simulink model "Md61Md62CalibSet"  (R2018b)
settings: Solver=FixedStepDiscrete  StartTime=0.0  StopTime=10.0  FixedStep=0.01  RelTol=1e-3
undefined symbols (not defined in the file or in its folder): KeSMSuFirstRwStBackPosDelta_Val, KeSMSuFirstRwStCushFoldPosDelta_Val, KeSMSuFirstRwStFwdBkwdPosDelta_Val, KeSMSuThrdRwCushFoldPosDelta_Val, KeSMSwAcsMd30PassStBkReclnUpwdDnwdPos1_Val, KeSMSwAcsMd30PassStBkReclnUpwdDnwdPos1Max_Val, KeSMSwAcsMd30PassStBkReclnUpwdDnwdPos1Min_Val, KeSMSwAcsMd30PassStFldUpwdDnwdPos1_Val, KeSMSwAcsMd30PassStFrwdBkwdPos1_Val, KeSMSwAcsMd30PassStFrwdBkwdPos1Max_Val, KeSMSwAcsMd30PassStFrwdBkwdPos1Min_Val, KeSMSwSeatBkLimitPos_Val, KeSMSwSeatBkLimitPosDelt_Val
libraries: StIsPosChkLib x2
(part 1 of 5)
settings Model: Creator=sn2xws  LastModifiedBy=sn55gm
settings Model: ModifiedHistory=|
  | 25.7.2 V3.13.0 新增Md61 Md62
  | 25.7.28 V3.13.1 BUG 1097903
  | 25.11.04 V3.13.2 副驾发送目标位置删除关于目标位置和limit的判断
settings DataIOCC: SaveFormat=StructureWithTime
settings OptimizationCC: DefaultParameterBehavior=Inlined  EnhancedBackFolding=on  PassReuseOutputArgsAs=Individual arguments  ZeroExternalMemoryAtStartup=off  ZeroInternalMemoryAtStartup=off  OptimizeBlockOrder=speed  DifferentSizesBufferReuse=on  OptimizationCustomize=off
settings DebuggingCC: ParameterTunabilityLossMsg=error
settings SFSimCC: MATLABDynamicMemAlloc=off
settings RTWCC: SystemTargetFile=autosar.tlc  GenCodeOnly=on  TemplateMakefile=ert_default_tmf  Description=AUTOSAR  GenerateReport=on  IncludeHyperlinkInReport=on  LaunchReport=on  GenerateTraceInfo=on  GenerateTraceReport=on  GenerateTraceReportSl=on  GenerateTraceReportSf=on  GenerateTraceReportEml=on
settings CodeAppCC: ForceParamTrailComments=on  IgnoreCustomStorageClasses=off  OperatorAnnotations=on  SimulinkDataObjDesc=on  SFDataObjDesc=on  InsertBlockDesc=on
settings STFCustomTargetCC: TargetLangStandard=C99 (ISO)  MultiwordLength=256  ParMdlRefBuildCompliant=on  CompOptLevelCompliant=on  IncludeMdlTerminateFcn=off  CombineOutputUpdateFcns=on  SuppressErrorStatus=on  ERTCustomFileBanners=on  SupportNonFinite=off  SupportComplex=off  SupportContinuousTime=off  SupportNonInlinedSFcns=off  RemoveResetFunc=on  MATLABClassNameForMDSCustomization=Simulink.SoftwareTarget.ERTCustomization  AutosarCompliant=on  UseToolchainInfoCompliant=on  LookupTableObjectStructAxisOrder=2,1,3,4,...  LUTObjectStructOrderEvenSpacing=Size,Table,Breakpoints  SystemTargetFile=autosar.tlc
settings ERTTargetCC: TargetLangStandard=C99 (ISO)  ConcurrentExecutionCompliant=off  IncludeMdlTerminateFcn=off  SuppressErrorStatus=on  SupportNonFinite=off  SupportComplex=off  ModelStepFunctionPrototypeControlCompliant=off  CPPClassGenCompliant=off  AutosarCompliant=on  LookupTableObjectStructAxisOrder=2,1,3,4,...  LUTObjectStructOrderEvenSpacing=Size,Table,Breakpoints  InlinedParameterPlacement=NonHierarchical  ERTCustomFileTemplate=example_file_process.tlc  ERTFilePackagingFormat=Compact

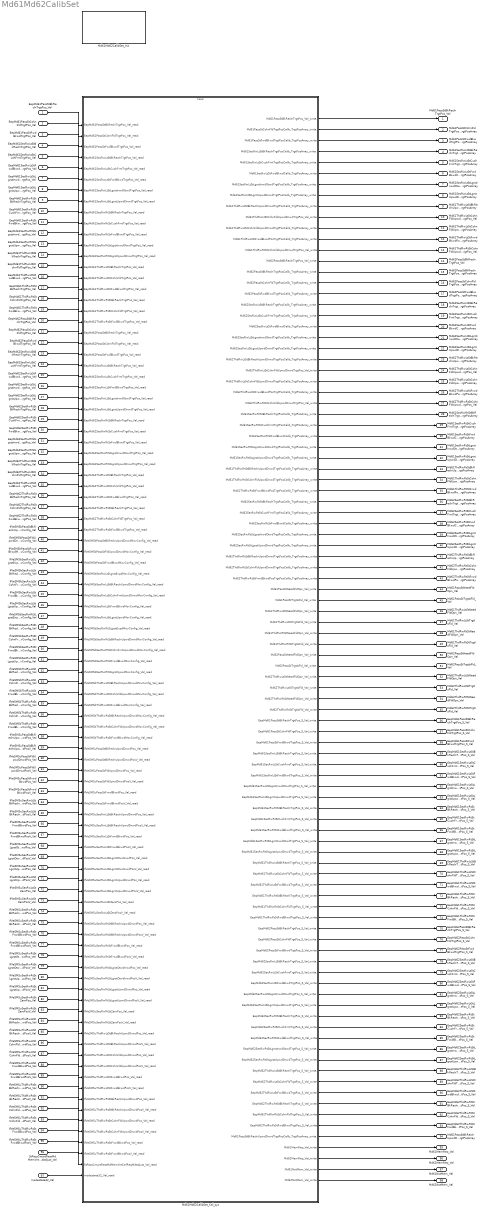
== system Md61Md62CalibSet ==
  EepMd61PassStBkReclnTrgtPos_Val : Inport  OutDataTypeStr=uint16  PortDimensions=1
  EepMd61PassStCshnFldTrgtPos_Val : Inport  Port=2  OutDataTypeStr=uint16  PortDimensions=1
  EepMd61PassStFwdBkwdTrgtPos_Val : Inport  Port=3  OutDataTypeStr=uint16  PortDimensions=1
  EepMd61SecRwLtStBkReclnTrgtPos_Val : Inport  Port=4  OutDataTypeStr=uint16  PortDimensions=1
  EepMd61SecRwLtStCushFrntTrgtPos_Val : Inport  Port=5  OutDataTypeStr=uint16  PortDimensions=1
  EepMd61SecRwLtStFwdBkwdTrgtPos_Val : Inport  Port=6  OutDataTypeStr=uint16  PortDimensions=1
  EepMd61SecRwLtStLgrstInwdOtwdTrgtPos_Val : Inport  Port=7  OutDataTypeStr=uint16  PortDimensions=1
  EepMd61SecRwLtStLgrstUpwdDnwdTrgtPos_Val : Inport  Port=8  OutDataTypeStr=uint16  PortDimensions=1
  EepMd61SecRwRtStBkReclnTrgtPos_Val : Inport  Port=9  OutDataTypeStr=uint16  PortDimensions=1
  EepMd61SecRwRtStCushFrntTrgtPos_Val : Inport  Port=10  OutDataTypeStr=uint16  PortDimensions=1
  EepMd61SecRwRtStFwdBkwdTrgtPos_Val : Inport  Port=11  OutDataTypeStr=uint16  PortDimensions=1
  EepMd61SecRwRtStLgrstInwdOtwdTrgtPos_Val : Inport  Port=12  OutDataTypeStr=uint16  PortDimensions=1
  EepMd61SecRwRtStLgrstUpwdDnwdTrgtPos_Val : Inport  Port=13  OutDataTypeStr=uint16  PortDimensions=1
  EepMd61ThdRwLtStBkReclnTrgtPos_Val : Inport  Port=14  OutDataTypeStr=uint16  PortDimensions=1
  EepMd61ThdRwLtStCshnFldTrgtPos_Val : Inport  Port=15  OutDataTypeStr=uint16  PortDimensions=1
  EepMd61ThdRwLtStFwdBkwdTrgtPos_Val : Inport  Port=16  OutDataTypeStr=uint16  PortDimensions=1
  EepMd61ThdRwRtStBkReclnTrgtPos_Val : Inport  Port=17  OutDataTypeStr=uint16  PortDimensions=1
  EepMd61ThdRwRtStCshnFldTrgtPos_Val : Inport  Port=18  OutDataTypeStr=uint16  PortDimensions=1
  EepMd61ThdRwRtStFwdBkwdTrgtPos_Val : Inport  Port=19  OutDataTypeStr=uint16  PortDimensions=1
  EepMd62PassStBkReclnTrgtPos_Val : Inport  Port=20  OutDataTypeStr=uint16  PortDimensions=1
  EepMd62PassStCshnFldTrgtPos_Val : Inport  Port=21  OutDataTypeStr=uint16  PortDimensions=1
  EepMd62PassStFwdBkwdTrgtPos_Val : Inport  Port=22  OutDataTypeStr=uint16  PortDimensions=1
  EepMd62SecRwLtStBkReclnTrgtPos_Val : Inport  Port=23  OutDataTypeStr=uint16  PortDimensions=1
  EepMd62SecRwLtStCushFrntTrgtPos_Val : Inport  Port=24  OutDataTypeStr=uint16  PortDimensions=1
  EepMd62SecRwLtStFwdBkwdTrgtPos_Val : Inport  Port=25  OutDataTypeStr=uint16  PortDimensions=1
  EepMd62SecRwLtStLgrstInwdOtwdTrgtPos_Val : Inport  Port=26  OutDataTypeStr=uint16  PortDimensions=1
  EepMd62SecRwLtStLgrstUpwdDnwdTrgtPos_Val : Inport  Port=27  OutDataTypeStr=uint16  PortDimensions=1
  EepMd62SecRwRtStBkReclnTrgtPos_Val : Inport  Port=28  OutDataTypeStr=uint16  PortDimensions=1
  EepMd62SecRwRtStCushFrntTrgtPos_Val : Inport  Port=29  OutDataTypeStr=uint16  PortDimensions=1
  EepMd62SecRwRtStFwdBkwdTrgtPos_Val : Inport  Port=30  OutDataTypeStr=uint16  PortDimensions=1
  EepMd62SecRwRtStLgrstInwdOtwdTrgtPos_Val : Inport  Port=31  OutDataTypeStr=uint16  PortDimensions=1
  EepMd62SecRwRtStLgrstUpwdDnwdTrgtPos_Val : Inport  Port=32  OutDataTypeStr=uint16  PortDimensions=1
  EepMd62ThdRwLtStBkReclnTrgtPos_Val : Inport  Port=33  OutDataTypeStr=uint16  PortDimensions=1
  EepMd62ThdRwLtStCshnFldTrgtPos_Val : Inport  Port=34  OutDataTypeStr=uint16  PortDimensions=1
  EepMd62ThdRwLtStFwdBkwdTrgtPos_Val : Inport  Port=35  OutDataTypeStr=uint16  PortDimensions=1
  EepMd62ThdRwRtStBkReclnTrgtPos_Val : Inport  Port=36  OutDataTypeStr=uint16  PortDimensions=1
  EepMd62ThdRwRtStCshnFldTrgtPos_Val : Inport  Port=37  OutDataTypeStr=uint16  PortDimensions=1
  EepMd62ThdRwRtStFwdBkwdTrgtPos_Val : Inport  Port=38  OutDataTypeStr=uint16  PortDimensions=1
  IfVeSMSbPassStBkReclnUpwdDnwdMovConfig_Val : Inport  Port=39  OutDataTypeStr=boolean  PortDimensions=1
  IfVeSMSbPassStFldUpwdDnwdMovConfig_Val : Inport  Port=40  OutDataTypeStr=boolean  PortDimensions=1
  IfVeSMSbPassStFrwdBkwdMovConfig_Val : Inport  Port=41  OutDataTypeStr=boolean  PortDimensions=1
  IfVeSMSbSecRwLtSLgrstExpdMovConfig_Val : Inport  Port=42  OutDataTypeStr=boolean  PortDimensions=1
  IfVeSMSbSecRwLtStBkReclnUpwdDnwdMovConfig_Val : Inport  Port=43  OutDataTypeStr=boolean  PortDimensions=1
  IfVeSMSbSecRwLtStCshnFrntUpwdDnwdMovConfig_Val : Inport  Port=44  OutDataTypeStr=boolean  PortDimensions=1
  IfVeSMSbSecRwLtStFrwdBkwdMovConfig_Val : Inport  Port=45  OutDataTypeStr=boolean  PortDimensions=1
  IfVeSMSbSecRwLtStLgrstUpwdMovConfig_Val : Inport  Port=46  OutDataTypeStr=boolean  PortDimensions=1
  IfVeSMSbSecRwRtSLgrstExpdMovConfig_Val : Inport  Port=47  OutDataTypeStr=boolean  PortDimensions=1
  IfVeSMSbSecRwRtStBkReclnUpwdDnwdMovConfig_Val : Inport  Port=48  OutDataTypeStr=boolean  PortDimensions=1
  IfVeSMSbSecRwRtStCshnFrntUpwdDnwdMovConfig_Val : Inport  Port=49  OutDataTypeStr=boolean  PortDimensions=1
  IfVeSMSbSecRwRtStFrwdBkwdMovConfig_Val : Inport  Port=50  OutDataTypeStr=boolean  PortDimensions=1
  IfVeSMSbSecRwRtStLgrstUpwdMovConfig_Val : Inport  Port=51  OutDataTypeStr=boolean  PortDimensions=1
  IfVeSMSbThdRwLtStBkReclnUpwdDnwdMovConfig_Val : Inport  Port=52  OutDataTypeStr=boolean  PortDimensions=1
  IfVeSMSbThdRwLtStCshnFldUpwdDnwdMovConfig_Val : Inport  Port=53  OutDataTypeStr=boolean  PortDimensions=1
  IfVeSMSbThdRwLtStFrwdBkwdMovConfig_Val : Inport  Port=54  OutDataTypeStr=boolean  PortDimensions=1
  IfVeSMSbThdRwRtStBkReclnUpwdDnwdMovConfig_Val : Inport  Port=55  OutDataTypeStr=boolean  PortDimensions=1
  IfVeSMSbThdRwRtStCshnFldUpwdDnwdMovConfig_Val : Inport  Port=56  OutDataTypeStr=boolean  PortDimensions=1
  IfVeSMSbThdRwRtStFrwdBkwdMovConfig_Val : Inport  Port=57  OutDataTypeStr=boolean  PortDimensions=1
  IfVeSMSuPassStBkReclnUpwdDnwdPos_Val : Inport  Port=58  OutDataTypeStr=uint16  PortDimensions=1
  IfVeSMSuPassStBkReclnUpwdDnwdPosV_Val : Inport  Port=59  OutDataTypeStr=boolean  PortDimensions=1
  IfVeSMSuPassStFldUpwdDnwdPos_Val : Inport  Port=60  OutDataTypeStr=uint16  PortDimensions=1
  IfVeSMSuPassStFldUpwdDnwdPosV_Val : Inport  Port=61  OutDataTypeStr=boolean  PortDimensions=1
  IfVeSMSuPassStFrwdBkwdPos_Val : Inport  Port=62  OutDataTypeStr=uint16  PortDimensions=1
  IfVeSMSuPassStFrwdBkwdPosV_Val : Inport  Port=63  OutDataTypeStr=boolean  PortDimensions=1
  IfVeSMSuSecRwLtStBkReclnUpwdDnwdPos_Val : Inport  Port=64  OutDataTypeStr=uint16  PortDimensions=1
  IfVeSMSuSecRwLtStBkReclnUpwdDnwdPosV_Val : Inport  Port=65  OutDataTypeStr=boolean  PortDimensions=1
  IfVeSMSuSecRwLtStFrwdBkwdPos_Val : Inport  Port=66  OutDataTypeStr=uint16  PortDimensions=1
  IfVeSMSuSecRwLtStFrwdBkwdPosV_Val : Inport  Port=67  OutDataTypeStr=boolean  PortDimensions=1
  IfVeSMSuSecRwLtStLgrstOtwdInwdPos_Val : Inport  Port=68  OutDataTypeStr=uint16  PortDimensions=1
  IfVeSMSuSecRwLtStLgrstOtwdInwdPosV_Val : Inport  Port=69  OutDataTypeStr=boolean  PortDimensions=1
  IfVeSMSuSecRwLtStLgrstUpwdDnwdPos_Val : Inport  Port=70  OutDataTypeStr=uint16  PortDimensions=1
  IfVeSMSuSecRwLtStLgrstUpwdDnwdPosV_Val : Inport  Port=71  OutDataTypeStr=boolean  PortDimensions=1
  IfVeSMSuSecRwLtStZeroPos_Val : Inport  Port=72  OutDataTypeStr=uint16  PortDimensions=1
  IfVeSMSuSecRwLtStZeroPosV_Val : Inport  Port=73  OutDataTypeStr=boolean  PortDimensions=1
  IfVeSMSuSecRwRtStBkReclnUpwdDnwdPos_Val : Inport  Port=74  OutDataTypeStr=uint16  PortDimensions=1
  IfVeSMSuSecRwRtStBkReclnUpwdDnwdPosV_Val : Inport  Port=75  OutDataTypeStr=boolean  PortDimensions=1
  IfVeSMSuSecRwRtStFrwdBkwdPos_Val : Inport  Port=76  OutDataTypeStr=uint16  PortDimensions=1
  IfVeSMSuSecRwRtStFrwdBkwdPosV_Val : Inport  Port=77  OutDataTypeStr=boolean  PortDimensions=1
  IfVeSMSuSecRwRtStLgrstOtwdInwdPos_Val : Inport  Port=78  OutDataTypeStr=uint16  PortDimensions=1
  IfVeSMSuSecRwRtStLgrstOtwdInwdPosV_Val : Inport  Port=79  OutDataTypeStr=boolean  PortDimensions=1
  IfVeSMSuSecRwRtStLgrstUpwdDnwdPos_Val : Inport  Port=80  OutDataTypeStr=uint16  PortDimensions=1
  IfVeSMSuSecRwRtStLgrstUpwdDnwdPosV_Val : Inport  Port=81  OutDataTypeStr=boolean  PortDimensions=1
  IfVeSMSuSecRwRtStZeroPos_Val : Inport  Port=82  OutDataTypeStr=uint16  PortDimensions=1
  IfVeSMSuSecRwRtStZeroPosV_Val : Inport  Port=83  OutDataTypeStr=boolean  PortDimensions=1
  IfVeSMSuThdRwLtStBkReclnUpwdDnwdPos_Val : Inport  Port=84  OutDataTypeStr=uint16  PortDimensions=1
  IfVeSMSuThdRwLtStBkReclnUpwdDnwdPosV_Val : Inport  Port=85  OutDataTypeStr=boolean  PortDimensions=1
  IfVeSMSuThdRwLtStCshnFldUpwdDnwdPos_Val : Inport  Port=86  OutDataTypeStr=uint16  PortDimensions=1
  IfVeSMSuThdRwLtStCshnFldUpwdDnwdPosV_Val : Inport  Port=87  OutDataTypeStr=boolean  PortDimensions=1
  IfVeSMSuThdRwLtStFrwdBkwdPos_Val : Inport  Port=88  OutDataTypeStr=uint16  PortDimensions=1
  IfVeSMSuThdRwLtStFrwdBkwdPosV_Val : Inport  Port=89  OutDataTypeStr=boolean  PortDimensions=1
  IfVeSMSuThdRwRtStBkReclnUpwdDnwdPos_Val : Inport  Port=90  OutDataTypeStr=uint16  PortDimensions=1
  IfVeSMSuThdRwRtStBkReclnUpwdDnwdPosV_Val : Inport  Port=91  OutDataTypeStr=boolean  PortDimensions=1
  IfVeSMSuThdRwRtStCshnFldUpwdDnwdPos_Val : Inport  Port=92  OutDataTypeStr=uint16  PortDimensions=1
  IfVeSMSuThdRwRtStCshnFldUpwdDnwdPosV_Val : Inport  Port=93  OutDataTypeStr=boolean  PortDimensions=1
  IfVeSMSuThdRwRtStFrwdBkwdPos_Val : Inport  Port=94  OutDataTypeStr=uint16  PortDimensions=1
  IfVeSMSuThdRwRtStFrwdBkwdPosV_Val : Inport  Port=95  OutDataTypeStr=boolean  PortDimensions=1
  StPassCmprtRestMdMemVirtCtrlReqMdadjust_Val : Inport  Port=96  OutDataTypeStr=uint8  PortDimensions=1
  modestate32_Val : Inport  Port=97  OutDataTypeStr=uint32  PortDimensions=1
  Md61Md62CalibSet_Cal_sys : Subsystem
  Md61Md62CalibSet_Init : Subsystem
  Md61PassStBkReclnTrgtPos_Val : Outport  OutDataTypeStr=uint16  PortDimensions=1
  Md61PassStCshnFldTrgtPosCalib_TrgtPosArray : Outport  Description=|  Port=2  OutDataTypeStr=uint16  PortDimensions=3
      | 0:Pos
      | 1:Max
      | 2:Min
  Md61PassStFwdBkwdTrgtPosCalib_TrgtPosArray : Outport  Description=|  Port=3  OutDataTypeStr=uint16  PortDimensions=3
      | 0:Pos
      | 1:Max
      | 2:Min
  Md61SecRwLtStBkReclnTrgtPosCalib_TrgtPosArray : Outport  Description=|  Port=4  OutDataTypeStr=uint16  PortDimensions=3
      | 0:Pos
      | 1:Max
      | 2:Min
  Md61SecRwLtStCushFrntTrgtPosCalib_TrgtPosArray : Outport  Description=|  Port=5  OutDataTypeStr=uint16  PortDimensions=3
      | 0:Pos
      | 1:Max
      | 2:Min
  Md61SecRwLtStFwdBkwdCalib_TrgtPosArray : Outport  Description=|  Port=6  OutDataTypeStr=uint16  PortDimensions=3
      | 0:Pos
      | 1:Max
      | 2:Min
  Md61SecRwLtStLgrstInwdOtwdTrgtPosCalib_TrgtPosArray : Outport  Description=|  Port=7  OutDataTypeStr=uint16  PortDimensions=3
      | 0:Pos
      | 1:Max
      | 2:Min
  Md61SecRwLtStLgrstUpwdDnwdTrgtPosCalib_TrgtPosArray : Outport  Description=|  Port=8  OutDataTypeStr=uint16  PortDimensions=3
      | 0:Pos
      | 1:Max
      | 2:Min
  Md61ThdRwLtStBkReclnUpwdDnwdTrgtPosCalib_TrgtPosArray : Outport  Description=|  Port=9  OutDataTypeStr=uint16  PortDimensions=3
      | 0:Pos
      | 1:Max
      | 2:Min
  Md61ThdRwLtStCshnFldUpwdDnwdTrgtPos_Val : Outport  Port=10  OutDataTypeStr=uint16  PortDimensions=1
  Md61ThdRwLtStCshnFldUpwdDnwdTrgtPosCalib_TrgtPosArray : Outport  Description=|  Port=11  OutDataTypeStr=uint16  PortDimensions=3
      | 0:Pos
      | 1:Max
      | 2:Min
  Md61ThdRwLtStFrwdBkwdPosTrgtPosCalib_TrgtPosArray : Outport  Description=|  Port=12  OutDataTypeStr=uint16  PortDimensions=3
      | 0:Pos
      | 1:Max
      | 2:Min
  Md61ThdRwRtStCshnFldUpwdDnwdTrgtPos_Val : Outport  Port=13  OutDataTypeStr=uint16  PortDimensions=1
  Md62PassStBkReclnTrgtPos_Val : Outport  Port=14  OutDataTypeStr=uint16  PortDimensions=1
  Md62PassStBkReclnTrgtPosCalib_TrgtPosArray : Outport  Description=|  Port=15  OutDataTypeStr=uint16  PortDimensions=3
      | 0:Pos
      | 1:Max
      | 2:Min
  Md62PassStCshnFldTrgtPosCalib_TrgtPosArray : Outport  Description=|  Port=16  OutDataTypeStr=uint16  PortDimensions=3
      | 0:Pos
      | 1:Max
      | 2:Min
  Md62PassStFwdBkwdTrgtPosCalib_TrgtPosArray : Outport  Description=|  Port=17  OutDataTypeStr=uint16  PortDimensions=3
      | 0:Pos
      | 1:Max
      | 2:Min
  Md62SecRwLtStBkReclnTrgtPosCalib_TrgtPosArray : Outport  Description=|  Port=18  OutDataTypeStr=uint16  PortDimensions=3
      | 0:Pos
      | 1:Max
      | 2:Min
  Md62SecRwLtStCushFrntTrgtPosCalib_TrgtPosArray : Outport  Description=|  Port=19  OutDataTypeStr=uint16  PortDimensions=3
      | 0:Pos
      | 1:Max
      | 2:Min
  Md62SecRwLtStFwdBkwdCalib_TrgtPosArray : Outport  Description=|  Port=20  OutDataTypeStr=uint16  PortDimensions=3
      | 0:Pos
      | 1:Max
      | 2:Min
  Md62SecRwLtStLgrstInwdOtwdTrgtPosCalib_TrgtPosArray : Outport  Description=|  Port=21  OutDataTypeStr=uint16  PortDimensions=3
      | 0:Pos
      | 1:Max
      | 2:Min
  Md62SecRwLtStLgrstUpwdDnwdTrgtPosCalib_TrgtPosArray : Outport  Description=|  Port=22  OutDataTypeStr=uint16  PortDimensions=3
      | 0:Pos
      | 1:Max
      | 2:Min
  Md62ThdRwLtStBkReclnUpwdDnwdTrgtPosCalib_TrgtPosArray : Outport  Description=|  Port=23  OutDataTypeStr=uint16  PortDimensions=3
      | 0:Pos
      | 1:Max
      | 2:Min
  Md62ThdRwLtStCshnFldUpwdDnwdTrgtPos_Val : Outport  Port=24  OutDataTypeStr=uint16  PortDimensions=1
  Md62ThdRwLtStCshnFldUpwdDnwdTrgtPosCalib_TrgtPosArray : Outport  Description=|  Port=25  OutDataTypeStr=uint16  PortDimensions=3
      | 0:Pos
      | 1:Max
      | 2:Min
  Md62ThdRwLtStFrwdBkwdPosTrgtPosCalib_TrgtPosArray : Outport  Description=|  Port=26  OutDataTypeStr=uint16  PortDimensions=3
      | 0:Pos
      | 1:Max
      | 2:Min
  Md62ThdRwRtStCshnFldUpwdDnwdTrgtPos_Val : Outport  Port=27  OutDataTypeStr=uint16  PortDimensions=1
  Md61SecRwRtStBkReclnTrgtPosCalib_TrgtPosArray : Outport  Description=|  Port=28  OutDataTypeStr=uint16  PortDimensions=3
      | 0:Pos
      | 1:Max
      | 2:Min
  Md61SecRwRtStCushFrntTrgtPosCalib_TrgtPosArray : Outport  Description=|  Port=29  OutDataTypeStr=uint16  PortDimensions=3
      | 0:Pos
      | 1:Max
      | 2:Min
  Md61SecRwRtStFwdBkwdCalib_TrgtPosArray : Outport  Description=|  Port=30  OutDataTypeStr=uint16  PortDimensions=3
      | 0:Pos
      | 1:Max
      | 2:Min
  Md61SecRwRtStLgrstInwdOtwdTrgtPosCalib_TrgtPosArray : Outport  Description=|  Port=31  OutDataTypeStr=uint16  PortDimensions=3
      | 0:Pos
      | 1:Max
      | 2:Min
  Md61SecRwRtStLgrstUpwdDnwdTrgtPosCalib_TrgtPosArray : Outport  Description=|  Port=32  OutDataTypeStr=uint16  PortDimensions=3
      | 0:Pos
      | 1:Max
      | 2:Min
  Md61ThdRwRtStBkReclnUpwdDnwdTrgtPosCalib_TrgtPosArray : Outport  Description=|  Port=33  OutDataTypeStr=uint16  PortDimensions=3
      | 0:Pos
      | 1:Max
      | 2:Min
  Md61ThdRwRtStCshnFldUpwdDnwdTrgtPosCalib_TrgtPosArray : Outport  Description=|  Port=34  OutDataTypeStr=uint16  PortDimensions=3
      | 0:Pos
      | 1:Max
      | 2:Min
  Md61ThdRwRtStFrwdBkwdPosTrgtPosCalib_TrgtPosArray : Outport  Description=|  Port=35  OutDataTypeStr=uint16  PortDimensions=3
      | 0:Pos
      | 1:Max
      | 2:Min
  Md62SecRwRtStBkReclnTrgtPosCalib_TrgtPosArray : Outport  Description=|  Port=36  OutDataTypeStr=uint16  PortDimensions=3
      | 0:Pos
      | 1:Max
      | 2:Min
  Md62SecRwRtStCushFrntTrgtPosCalib_TrgtPosArray : Outport  Description=|  Port=37  OutDataTypeStr=uint16  PortDimensions=3
      | 0:Pos
      | 1:Max
      | 2:Min
  Md62SecRwRtStFwdBkwdCalib_TrgtPosArray : Outport  Description=|  Port=38  OutDataTypeStr=uint16  PortDimensions=3
      | 0:Pos
      | 1:Max
      | 2:Min
  Md62SecRwRtStLgrstInwdOtwdTrgtPosCalib_TrgtPosArray : Outport  Description=|  Port=39  OutDataTypeStr=uint16  PortDimensions=3
      | 0:Pos
      | 1:Max
      | 2:Min
  Md62SecRwRtStLgrstUpwdDnwdTrgtPosCalib_TrgtPosArray : Outport  Description=|  Port=40  OutDataTypeStr=uint16  PortDimensions=3
      | 0:Pos
      | 1:Max
      | 2:Min
  Md62ThdRwRtStBkReclnUpwdDnwdTrgtPosCalib_TrgtPosArray : Outport  Description=|  Port=41  OutDataTypeStr=uint16  PortDimensions=3
      | 0:Pos
      | 1:Max
      | 2:Min
  Md62ThdRwRtStCshnFldUpwdDnwdTrgtPosCalib_TrgtPosArray : Outport  Description=|  Port=42  OutDataTypeStr=uint16  PortDimensions=3
      | 0:Pos
      | 1:Max
      | 2:Min
  Md62ThdRwRtStFrwdBkwdPosTrgtPosCalib_TrgtPosArray : Outport  Description=|  Port=43  OutDataTypeStr=uint16  PortDimensions=3
      | 0:Pos
      | 1:Max
      | 2:Min
  Md61PassStNeedFldOpn_Val : Outport  Port=44  OutDataTypeStr=boolean  PortDimensions=1
  Md61PassStTrgtIsFld_Val : Outport  Port=45  OutDataTypeStr=boolean  PortDimensions=1
  Md61ThdRwLtStNeedFldOpn_Val : Outport  Port=46  OutDataTypeStr=boolean  PortDimensions=1
  Md61ThdRwLtStTrgtIsFld_Val : Outport  Port=47  OutDataTypeStr=boolean  PortDimensions=1
  Md61ThdRwRtStNeedFldOpn_Val : Outport  Port=48  OutDataTypeStr=boolean  PortDimensions=1
  Md61ThdRwRtStTrgtIsFld_Val : Outport  Port=49  OutDataTypeStr=boolean  PortDimensions=1
  Md62PassStNeedFldOpn_Val : Outport  Port=50  OutDataTypeStr=boolean  PortDimensions=1
  Md62PassStTrgtIsFld_Val : Outport  Port=51  OutDataTypeStr=boolean  PortDimensions=1
  Md62ThdRwLtStNeedFldOpn_Val : Outport  Port=52  OutDataTypeStr=boolean  PortDimensions=1
  Md62ThdRwLtStTrgtIsFld_Val : Outport  Port=53  OutDataTypeStr=boolean  PortDimensions=1
  Md62ThdRwRtStNeedFldOpn_Val : Outport  Port=54  OutDataTypeStr=boolean  PortDimensions=1
  Md62ThdRwRtStTrgtIsFld_Val : Outport  Port=55  OutDataTypeStr=boolean  PortDimensions=1
  EepMd61PassStBkReclnTrgtPos_S_Val : Outport  Port=56  OutDataTypeStr=uint16  PortDimensions=1
  EepMd61PassStCshnFldTrgtPos_S_Val : Outport  Port=57  OutDataTypeStr=uint16  PortDimensions=1
  EepMd61PassStFwdBkwdTrgtPos_S_Val : Outport  Port=58  OutDataTypeStr=uint16  PortDimensions=1
  EepMd61SecRwLtStBkReclnTrgtPos_S_Val : Outport  Port=59  OutDataTypeStr=uint16  PortDimensions=1
  EepMd61SecRwLtStCushFrntTrgtPos_S_Val : Outport  Port=60  OutDataTypeStr=uint16  PortDimensions=1
  EepMd61SecRwLtStFwdBkwdTrgtPos_S_Val : Outport  Port=61  OutDataTypeStr=uint16  PortDimensions=1
  EepMd61SecRwLtStLgrstInwdOtwdTrgtPos_S_Val : Outport  Port=62  OutDataTypeStr=uint16  PortDimensions=1
  EepMd61SecRwLtStLgrstUpwdDnwdTrgtPos_S_Val : Outport  Port=63  OutDataTypeStr=uint16  PortDimensions=1
  EepMd61SecRwRtStBkReclnTrgtPos_S_Val : Outport  Port=64  OutDataTypeStr=uint16  PortDimensions=1
  EepMd61SecRwRtStCushFrntTrgtPos_S_Val : Outport  Port=65  OutDataTypeStr=uint16  PortDimensions=1
  EepMd61SecRwRtStFwdBkwdTrgtPos_S_Val : Outport  Port=66  OutDataTypeStr=uint16  PortDimensions=1
  EepMd61SecRwRtStLgrstInwdOtwdTrgtPos_S_Val : Outport  Port=67  OutDataTypeStr=uint16  PortDimensions=1
  EepMd61SecRwRtStLgrstUpwdDnwdTrgtPos_S_Val : Outport  Port=68  OutDataTypeStr=uint16  PortDimensions=1
  EepMd61ThdRwLtStBkReclnTrgtPos_S_Val : Outport  Port=69  OutDataTypeStr=uint16  PortDimensions=1
  EepMd61ThdRwLtStCshnFldTrgtPos_S_Val : Outport  Port=70  OutDataTypeStr=uint16  PortDimensions=1
  EepMd61ThdRwLtStFwdBkwdTrgtPos_S_Val : Outport  Port=71  OutDataTypeStr=uint16  PortDimensions=1
  EepMd61ThdRwRtStBkReclnTrgtPos_S_Val : Outport  Port=72  OutDataTypeStr=uint16  PortDimensions=1
  EepMd61ThdRwRtStCshnFldTrgtPos_S_Val : Outport  Port=73  OutDataTypeStr=uint16  PortDimensions=1
  EepMd61ThdRwRtStFwdBkwdTrgtPos_S_Val : Outport  Port=74  OutDataTypeStr=uint16  PortDimensions=1
  EepMd62PassStBkReclnTrgtPos_S_Val : Outport  Port=75  OutDataTypeStr=uint16  PortDimensions=1
  EepMd62PassStCshnFldTrgtPos_S_Val : Outport  Port=76  OutDataTypeStr=uint16  PortDimensions=1
  EepMd62PassStFwdBkwdTrgtPos_S_Val : Outport  Port=77  OutDataTypeStr=uint16  PortDimensions=1
  EepMd62SecRwLtStBkReclnTrgtPos_S_Val : Outport  Port=78  OutDataTypeStr=uint16  PortDimensions=1
  EepMd62SecRwLtStCushFrntTrgtPos_S_Val : Outport  Port=79  OutDataTypeStr=uint16  PortDimensions=1
  EepMd62SecRwLtStFwdBkwdTrgtPos_S_Val : Outport  Port=80  OutDataTypeStr=uint16  PortDimensions=1
  EepMd62SecRwLtStLgrstInwdOtwdTrgtPos_S_Val : Outport  Port=81  OutDataTypeStr=uint16  PortDimensions=1
  EepMd62SecRwLtStLgrstUpwdDnwdTrgtPos_S_Val : Outport  Port=82  OutDataTypeStr=uint16  PortDimensions=1
  EepMd62SecRwRtStBkReclnTrgtPos_S_Val : Outport  Port=83  OutDataTypeStr=uint16  PortDimensions=1
  EepMd62SecRwRtStCushFrntTrgtPos_S_Val : Outport  Port=84  OutDataTypeStr=uint16  PortDimensions=1
  EepMd62SecRwRtStFwdBkwdTrgtPos_S_Val : Outport  Port=85  OutDataTypeStr=uint16  PortDimensions=1
  EepMd62SecRwRtStLgrstInwdOtwdTrgtPos_S_Val : Outport  Port=86  OutDataTypeStr=uint16  PortDimensions=1
  EepMd62SecRwRtStLgrstUpwdDnwdTrgtPos_S_Val : Outport  Port=87  OutDataTypeStr=uint16  PortDimensions=1
  EepMd62ThdRwLtStBkReclnTrgtPos_S_Val : Outport  Port=88  OutDataTypeStr=uint16  PortDimensions=1
  EepMd62ThdRwLtStCshnFldTrgtPos_S_Val : Outport  Port=89  OutDataTypeStr=uint16  PortDimensions=1
  EepMd62ThdRwLtStFwdBkwdTrgtPos_S_Val : Outport  Port=90  OutDataTypeStr=uint16  PortDimensions=1
  EepMd62ThdRwRtStBkReclnTrgtPos_S_Val : Outport  Port=91  OutDataTypeStr=uint16  PortDimensions=1
  EepMd62ThdRwRtStCshnFldTrgtPos_S_Val : Outport  Port=92  OutDataTypeStr=uint16  PortDimensions=1
  EepMd62ThdRwRtStFwdBkwdTrgtPos_S_Val : Outport  Port=93  OutDataTypeStr=uint16  PortDimensions=1
  Md61PassStBkReclnUpwdDnwdTrgtPosCalib_TrgtPosArray : Outport  Description=|  Port=94  OutDataTypeStr=uint16  PortDimensions=3
      | 0:Pos
      | 1:Max
      | 2:Min
  Md61MemReq_Val : Outport  Port=95  OutDataTypeStr=boolean  PortDimensions=1
  Md62MemReq_Val : Outport  Port=96  OutDataTypeStr=boolean  PortDimensions=1
  Md61NotMem_Val : Outport  Port=97  OutDataTypeStr=boolean  PortDimensions=1
  Md62NotMem_Val : Outport  Port=98  OutDataTypeStr=boolean  PortDimensions=1
  wires:
  EepMd61PassStBkReclnTrgtPos_Val/1 -> Md61Md62CalibSet_Cal_sys/1(EepMd61PassStBkReclnTrgtPos_Val_read)
  EepMd61PassStCshnFldTrgtPos_Val/1 -> Md61Md62CalibSet_Cal_sys/2(EepMd61PassStCshnFldTrgtPos_Val_read)
  EepMd61PassStFwdBkwdTrgtPos_Val/1 -> Md61Md62CalibSet_Cal_sys/3(EepMd61PassStFwdBkwdTrgtPos_Val_read)
  EepMd61SecRwLtStBkReclnTrgtPos_Val/1 -> Md61Md62CalibSet_Cal_sys/4(EepMd61SecRwLtStBkReclnTrgtPos_Val_read)
  EepMd61SecRwLtStCushFrntTrgtPos_Val/1 -> Md61Md62CalibSet_Cal_sys/5(EepMd61SecRwLtStCushFrntTrgtPos_Val_read)
  EepMd61SecRwLtStFwdBkwdTrgtPos_Val/1 -> Md61Md62CalibSet_Cal_sys/6(EepMd61SecRwLtStFwdBkwdTrgtPos_Val_read)
  EepMd61SecRwLtStLgrstInwdOtwdTrgtPos_Val/1 -> Md61Md62CalibSet_Cal_sys/7(EepMd61SecRwLtStLgrstInwdOtwdTrgtPos_Val_read)
  EepMd61SecRwLtStLgrstUpwdDnwdTrgtPos_Val/1 -> Md61Md62CalibSet_Cal_sys/8(EepMd61SecRwLtStLgrstUpwdDnwdTrgtPos_Val_read)
  EepMd61SecRwRtStBkReclnTrgtPos_Val/1 -> Md61Md62CalibSet_Cal_sys/9(EepMd61SecRwRtStBkReclnTrgtPos_Val_read)
  EepMd61SecRwRtStCushFrntTrgtPos_Val/1 -> Md61Md62CalibSet_Cal_sys/10(EepMd61SecRwRtStCushFrntTrgtPos_Val_read)
  EepMd61SecRwRtStFwdBkwdTrgtPos_Val/1 -> Md61Md62CalibSet_Cal_sys/11(EepMd61SecRwRtStFwdBkwdTrgtPos_Val_read)
  EepMd61SecRwRtStLgrstInwdOtwdTrgtPos_Val/1 -> Md61Md62CalibSet_Cal_sys/12(EepMd61SecRwRtStLgrstInwdOtwdTrgtPos_Val_read)
  EepMd61SecRwRtStLgrstUpwdDnwdTrgtPos_Val/1 -> Md61Md62CalibSet_Cal_sys/13(EepMd61SecRwRtStLgrstUpwdDnwdTrgtPos_Val_read)
  EepMd61ThdRwLtStBkReclnTrgtPos_Val/1 -> Md61Md62CalibSet_Cal_sys/14(EepMd61ThdRwLtStBkReclnTrgtPos_Val_read)
  EepMd61ThdRwLtStCshnFldTrgtPos_Val/1 -> Md61Md62CalibSet_Cal_sys/15(EepMd61ThdRwLtStCshnFldTrgtPos_Val_read)
  EepMd61ThdRwLtStFwdBkwdTrgtPos_Val/1 -> Md61Md62CalibSet_Cal_sys/16(EepMd61ThdRwLtStFwdBkwdTrgtPos_Val_read)
  EepMd61ThdRwRtStBkReclnTrgtPos_Val/1 -> Md61Md62CalibSet_Cal_sys/17(EepMd61ThdRwRtStBkReclnTrgtPos_Val_read)
  EepMd61ThdRwRtStCshnFldTrgtPos_Val/1 -> Md61Md62CalibSet_Cal_sys/18(EepMd61ThdRwRtStCshnFldTrgtPos_Val_read)
  EepMd61ThdRwRtStFwdBkwdTrgtPos_Val/1 -> Md61Md62CalibSet_Cal_sys/19(EepMd61ThdRwRtStFwdBkwdTrgtPos_Val_read)
  EepMd62PassStBkReclnTrgtPos_Val/1 -> Md61Md62CalibSet_Cal_sys/20(EepMd62PassStBkReclnTrgtPos_Val_read)
  EepMd62PassStCshnFldTrgtPos_Val/1 -> Md61Md62CalibSet_Cal_sys/21(EepMd62PassStCshnFldTrgtPos_Val_read)
  EepMd62PassStFwdBkwdTrgtPos_Val/1 -> Md61Md62CalibSet_Cal_sys/22(EepMd62PassStFwdBkwdTrgtPos_Val_read)
  EepMd62SecRwLtStBkReclnTrgtPos_Val/1 -> Md61Md62CalibSet_Cal_sys/23(EepMd62SecRwLtStBkReclnTrgtPos_Val_read)
  EepMd62SecRwLtStCushFrntTrgtPos_Val/1 -> Md61Md62CalibSet_Cal_sys/24(EepMd62SecRwLtStCushFrntTrgtPos_Val_read)
  EepMd62SecRwLtStFwdBkwdTrgtPos_Val/1 -> Md61Md62CalibSet_Cal_sys/25(EepMd62SecRwLtStFwdBkwdTrgtPos_Val_read)
  EepMd62SecRwLtStLgrstInwdOtwdTrgtPos_Val/1 -> Md61Md62CalibSet_Cal_sys/26(EepMd62SecRwLtStLgrstInwdOtwdTrgtPos_Val_read)
  EepMd62SecRwLtStLgrstUpwdDnwdTrgtPos_Val/1 -> Md61Md62CalibSet_Cal_sys/27(EepMd62SecRwLtStLgrstUpwdDnwdTrgtPos_Val_read)
  EepMd62SecRwRtStBkReclnTrgtPos_Val/1 -> Md61Md62CalibSet_Cal_sys/28(EepMd62SecRwRtStBkReclnTrgtPos_Val_read)
  EepMd62SecRwRtStCushFrntTrgtPos_Val/1 -> Md61Md62CalibSet_Cal_sys/29(EepMd62SecRwRtStCushFrntTrgtPos_Val_read)
  EepMd62SecRwRtStFwdBkwdTrgtPos_Val/1 -> Md61Md62CalibSet_Cal_sys/30(EepMd62SecRwRtStFwdBkwdTrgtPos_Val_read)
  EepMd62SecRwRtStLgrstInwdOtwdTrgtPos_Val/1 -> Md61Md62CalibSet_Cal_sys/31(EepMd62SecRwRtStLgrstInwdOtwdTrgtPos_Val_read)
  EepMd62SecRwRtStLgrstUpwdDnwdTrgtPos_Val/1 -> Md61Md62CalibSet_Cal_sys/32(EepMd62SecRwRtStLgrstUpwdDnwdTrgtPos_Val_read)
  EepMd62ThdRwLtStBkReclnTrgtPos_Val/1 -> Md61Md62CalibSet_Cal_sys/33(EepMd62ThdRwLtStBkReclnTrgtPos_Val_read)
  EepMd62ThdRwLtStCshnFldTrgtPos_Val/1 -> Md61Md62CalibSet_Cal_sys/34(EepMd62ThdRwLtStCshnFldTrgtPos_Val_read)
  EepMd62ThdRwLtStFwdBkwdTrgtPos_Val/1 -> Md61Md62CalibSet_Cal_sys/35(EepMd62ThdRwLtStFwdBkwdTrgtPos_Val_read)
  EepMd62ThdRwRtStBkReclnTrgtPos_Val/1 -> Md61Md62CalibSet_Cal_sys/36(EepMd62ThdRwRtStBkReclnTrgtPos_Val_read)
  EepMd62ThdRwRtStCshnFldTrgtPos_Val/1 -> Md61Md62CalibSet_Cal_sys/37(EepMd62ThdRwRtStCshnFldTrgtPos_Val_read)
  EepMd62ThdRwRtStFwdBkwdTrgtPos_Val/1 -> Md61Md62CalibSet_Cal_sys/38(EepMd62ThdRwRtStFwdBkwdTrgtPos_Val_read)
  IfVeSMSbPassStBkReclnUpwdDnwdMovConfig_Val/1 -> Md61Md62CalibSet_Cal_sys/39(IfVeSMSbPassStBkReclnUpwdDnwdMovConfig_Val_read)
  IfVeSMSbPassStFldUpwdDnwdMovConfig_Val/1 -> Md61Md62CalibSet_Cal_sys/40(IfVeSMSbPassStFldUpwdDnwdMovConfig_Val_read)
  IfVeSMSbPassStFrwdBkwdMovConfig_Val/1 -> Md61Md62CalibSet_Cal_sys/41(IfVeSMSbPassStFrwdBkwdMovConfig_Val_read)
  IfVeSMSbSecRwLtSLgrstExpdMovConfig_Val/1 -> Md61Md62CalibSet_Cal_sys/42(IfVeSMSbSecRwLtSLgrstExpdMovConfig_Val_read)
  IfVeSMSbSecRwLtStBkReclnUpwdDnwdMovConfig_Val/1 -> Md61Md62CalibSet_Cal_sys/43(IfVeSMSbSecRwLtStBkReclnUpwdDnwdMovConfig_Val_read)
  IfVeSMSbSecRwLtStCshnFrntUpwdDnwdMovConfig_Val/1 -> Md61Md62CalibSet_Cal_sys/44(IfVeSMSbSecRwLtStCshnFrntUpwdDnwdMovConfig_Val_read)
  IfVeSMSbSecRwLtStFrwdBkwdMovConfig_Val/1 -> Md61Md62CalibSet_Cal_sys/45(IfVeSMSbSecRwLtStFrwdBkwdMovConfig_Val_read)
  IfVeSMSbSecRwLtStLgrstUpwdMovConfig_Val/1 -> Md61Md62CalibSet_Cal_sys/46(IfVeSMSbSecRwLtStLgrstUpwdMovConfig_Val_read)
  IfVeSMSbSecRwRtSLgrstExpdMovConfig_Val/1 -> Md61Md62CalibSet_Cal_sys/47(IfVeSMSbSecRwRtSLgrstExpdMovConfig_Val_read)
  IfVeSMSbSecRwRtStBkReclnUpwdDnwdMovConfig_Val/1 -> Md61Md62CalibSet_Cal_sys/48(IfVeSMSbSecRwRtStBkReclnUpwdDnwdMovConfig_Val_read)
  IfVeSMSbSecRwRtStCshnFrntUpwdDnwdMovConfig_Val/1 -> Md61Md62CalibSet_Cal_sys/49(IfVeSMSbSecRwRtStCshnFrntUpwdDnwdMovConfig_Val_read)
  IfVeSMSbSecRwRtStFrwdBkwdMovConfig_Val/1 -> Md61Md62CalibSet_Cal_sys/50(IfVeSMSbSecRwRtStFrwdBkwdMovConfig_Val_read)
  IfVeSMSbSecRwRtStLgrstUpwdMovConfig_Val/1 -> Md61Md62CalibSet_Cal_sys/51(IfVeSMSbSecRwRtStLgrstUpwdMovConfig_Val_read)
  IfVeSMSbThdRwLtStBkReclnUpwdDnwdMovConfig_Val/1 -> Md61Md62CalibSet_Cal_sys/52(IfVeSMSbThdRwLtStBkReclnUpwdDnwdMovConfig_Val_read)
  IfVeSMSbThdRwLtStCshnFldUpwdDnwdMovConfig_Val/1 -> Md61Md62CalibSet_Cal_sys/53(IfVeSMSbThdRwLtStCshnFldUpwdDnwdMovConfig_Val_read)
  IfVeSMSbThdRwLtStFrwdBkwdMovConfig_Val/1 -> Md61Md62CalibSet_Cal_sys/54(IfVeSMSbThdRwLtStFrwdBkwdMovConfig_Val_read)
  IfVeSMSbThdRwRtStBkReclnUpwdDnwdMovConfig_Val/1 -> Md61Md62CalibSet_Cal_sys/55(IfVeSMSbThdRwRtStBkReclnUpwdDnwdMovConfig_Val_read)
  IfVeSMSbThdRwRtStCshnFldUpwdDnwdMovConfig_Val/1 -> Md61Md62CalibSet_Cal_sys/56(IfVeSMSbThdRwRtStCshnFldUpwdDnwdMovConfig_Val_read)
  IfVeSMSbThdRwRtStFrwdBkwdMovConfig_Val/1 -> Md61Md62CalibSet_Cal_sys/57(IfVeSMSbThdRwRtStFrwdBkwdMovConfig_Val_read)
  IfVeSMSuPassStBkReclnUpwdDnwdPos_Val/1 -> Md61Md62CalibSet_Cal_sys/58(IfVeSMSuPassStBkReclnUpwdDnwdPos_Val_read)
  IfVeSMSuPassStBkReclnUpwdDnwdPosV_Val/1 -> Md61Md62CalibSet_Cal_sys/59(IfVeSMSuPassStBkReclnUpwdDnwdPosV_Val_read)
  IfVeSMSuPassStFldUpwdDnwdPos_Val/1 -> Md61Md62CalibSet_Cal_sys/60(IfVeSMSuPassStFldUpwdDnwdPos_Val_read)
  IfVeSMSuPassStFldUpwdDnwdPosV_Val/1 -> Md61Md62CalibSet_Cal_sys/61(IfVeSMSuPassStFldUpwdDnwdPosV_Val_read)
  IfVeSMSuPassStFrwdBkwdPos_Val/1 -> Md61Md62CalibSet_Cal_sys/62(IfVeSMSuPassStFrwdBkwdPos_Val_read)
  IfVeSMSuPassStFrwdBkwdPosV_Val/1 -> Md61Md62CalibSet_Cal_sys/63(IfVeSMSuPassStFrwdBkwdPosV_Val_read)
  IfVeSMSuSecRwLtStBkReclnUpwdDnwdPos_Val/1 -> Md61Md62CalibSet_Cal_sys/64(IfVeSMSuSecRwLtStBkReclnUpwdDnwdPos_Val_read)
  IfVeSMSuSecRwLtStBkReclnUpwdDnwdPosV_Val/1 -> Md61Md62CalibSet_Cal_sys/65(IfVeSMSuSecRwLtStBkReclnUpwdDnwdPosV_Val_read)
  IfVeSMSuSecRwLtStFrwdBkwdPos_Val/1 -> Md61Md62CalibSet_Cal_sys/66(IfVeSMSuSecRwLtStFrwdBkwdPos_Val_read)
  IfVeSMSuSecRwLtStFrwdBkwdPosV_Val/1 -> Md61Md62CalibSet_Cal_sys/67(IfVeSMSuSecRwLtStFrwdBkwdPosV_Val_read)
  IfVeSMSuSecRwLtStLgrstOtwdInwdPos_Val/1 -> Md61Md62CalibSet_Cal_sys/68(IfVeSMSuSecRwLtStLgrstOtwdInwdPos_Val_read)
  IfVeSMSuSecRwLtStLgrstOtwdInwdPosV_Val/1 -> Md61Md62CalibSet_Cal_sys/69(IfVeSMSuSecRwLtStLgrstOtwdInwdPosV_Val_read)
  IfVeSMSuSecRwLtStLgrstUpwdDnwdPos_Val/1 -> Md61Md62CalibSet_Cal_sys/70(IfVeSMSuSecRwLtStLgrstUpwdDnwdPos_Val_read)
  IfVeSMSuSecRwLtStLgrstUpwdDnwdPosV_Val/1 -> Md61Md62CalibSet_Cal_sys/71(IfVeSMSuSecRwLtStLgrstUpwdDnwdPosV_Val_read)
  IfVeSMSuSecRwLtStZeroPos_Val/1 -> Md61Md62CalibSet_Cal_sys/72(IfVeSMSuSecRwLtStZeroPos_Val_read)
  IfVeSMSuSecRwLtStZeroPosV_Val/1 -> Md61Md62CalibSet_Cal_sys/73(IfVeSMSuSecRwLtStZeroPosV_Val_read)
  IfVeSMSuSecRwRtStBkReclnUpwdDnwdPos_Val/1 -> Md61Md62CalibSet_Cal_sys/74(IfVeSMSuSecRwRtStBkReclnUpwdDnwdPos_Val_read)
  IfVeSMSuSecRwRtStBkReclnUpwdDnwdPosV_Val/1 -> Md61Md62CalibSet_Cal_sys/75(IfVeSMSuSecRwRtStBkReclnUpwdDnwdPosV_Val_read)
  IfVeSMSuSecRwRtStFrwdBkwdPos_Val/1 -> Md61Md62CalibSet_Cal_sys/76(IfVeSMSuSecRwRtStFrwdBkwdPos_Val_read)
  IfVeSMSuSecRwRtStFrwdBkwdPosV_Val/1 -> Md61Md62CalibSet_Cal_sys/77(IfVeSMSuSecRwRtStFrwdBkwdPosV_Val_read)
  IfVeSMSuSecRwRtStLgrstOtwdInwdPos_Val/1 -> Md61Md62CalibSet_Cal_sys/78(IfVeSMSuSecRwRtStLgrstOtwdInwdPos_Val_read)
  IfVeSMSuSecRwRtStLgrstOtwdInwdPosV_Val/1 -> Md61Md62CalibSet_Cal_sys/79(IfVeSMSuSecRwRtStLgrstOtwdInwdPosV_Val_read)
  IfVeSMSuSecRwRtStLgrstUpwdDnwdPos_Val/1 -> Md61Md62CalibSet_Cal_sys/80(IfVeSMSuSecRwRtStLgrstUpwdDnwdPos_Val_read)
  IfVeSMSuSecRwRtStLgrstUpwdDnwdPosV_Val/1 -> Md61Md62CalibSet_Cal_sys/81(IfVeSMSuSecRwRtStLgrstUpwdDnwdPosV_Val_read)
  IfVeSMSuSecRwRtStZeroPos_Val/1 -> Md61Md62CalibSet_Cal_sys/82(IfVeSMSuSecRwRtStZeroPos_Val_read)
  IfVeSMSuSecRwRtStZeroPosV_Val/1 -> Md61Md62CalibSet_Cal_sys/83(IfVeSMSuSecRwRtStZeroPosV_Val_read)
  IfVeSMSuThdRwLtStBkReclnUpwdDnwdPos_Val/1 -> Md61Md62CalibSet_Cal_sys/84(IfVeSMSuThdRwLtStBkReclnUpwdDnwdPos_Val_read)
  IfVeSMSuThdRwLtStBkReclnUpwdDnwdPosV_Val/1 -> Md61Md62CalibSet_Cal_sys/85(IfVeSMSuThdRwLtStBkReclnUpwdDnwdPosV_Val_read)
  IfVeSMSuThdRwLtStCshnFldUpwdDnwdPos_Val/1 -> Md61Md62CalibSet_Cal_sys/86(IfVeSMSuThdRwLtStCshnFldUpwdDnwdPos_Val_read)
  IfVeSMSuThdRwLtStCshnFldUpwdDnwdPosV_Val/1 -> Md61Md62CalibSet_Cal_sys/87(IfVeSMSuThdRwLtStCshnFldUpwdDnwdPosV_Val_read)
  IfVeSMSuThdRwLtStFrwdBkwdPos_Val/1 -> Md61Md62CalibSet_Cal_sys/88(IfVeSMSuThdRwLtStFrwdBkwdPos_Val_read)
  IfVeSMSuThdRwLtStFrwdBkwdPosV_Val/1 -> Md61Md62CalibSet_Cal_sys/89(IfVeSMSuThdRwLtStFrwdBkwdPosV_Val_read)
  IfVeSMSuThdRwRtStBkReclnUpwdDnwdPos_Val/1 -> Md61Md62CalibSet_Cal_sys/90(IfVeSMSuThdRwRtStBkReclnUpwdDnwdPos_Val_read)
  IfVeSMSuThdRwRtStBkReclnUpwdDnwdPosV_Val/1 -> Md61Md62CalibSet_Cal_sys/91(IfVeSMSuThdRwRtStBkReclnUpwdDnwdPosV_Val_read)
  IfVeSMSuThdRwRtStCshnFldUpwdDnwdPos_Val/1 -> Md61Md62CalibSet_Cal_sys/92(IfVeSMSuThdRwRtStCshnFldUpwdDnwdPos_Val_read)
  IfVeSMSuThdRwRtStCshnFldUpwdDnwdPosV_Val/1 -> Md61Md62CalibSet_Cal_sys/93(IfVeSMSuThdRwRtStCshnFldUpwdDnwdPosV_Val_read)
  IfVeSMSuThdRwRtStFrwdBkwdPos_Val/1 -> Md61Md62CalibSet_Cal_sys/94(IfVeSMSuThdRwRtStFrwdBkwdPos_Val_read)
  IfVeSMSuThdRwRtStFrwdBkwdPosV_Val/1 -> Md61Md62CalibSet_Cal_sys/95(IfVeSMSuThdRwRtStFrwdBkwdPosV_Val_read)
  StPassCmprtRestMdMemVirtCtrlReqMdadjust_Val/1 -> Md61Md62CalibSet_Cal_sys/96(StPassCmprtRestMdMemVirtCtrlReqMdadjust_Val_read)
  Md61Md62CalibSet_Cal_sys/1(Md61PassStBkReclnTrgtPos_Val_write) -> Md61PassStBkReclnTrgtPos_Val/1
  Md61Md62CalibSet_Cal_sys/2(Md61PassStCshnFldTrgtPosCalib_TrgtPosArray_write) -> Md61PassStCshnFldTrgtPosCalib_TrgtPosArray/1
  Md61Md62CalibSet_Cal_sys/3(Md61PassStFwdBkwdTrgtPosCalib_TrgtPosArray_write) -> Md61PassStFwdBkwdTrgtPosCalib_TrgtPosArray/1
  Md61Md62CalibSet_Cal_sys/4(Md61SecRwLtStBkReclnTrgtPosCalib_TrgtPosArray_write) -> Md61SecRwLtStBkReclnTrgtPosCalib_TrgtPosArray/1
  Md61Md62CalibSet_Cal_sys/5(Md61SecRwLtStCushFrntTrgtPosCalib_TrgtPosArray_write) -> Md61SecRwLtStCushFrntTrgtPosCalib_TrgtPosArray/1
  Md61Md62CalibSet_Cal_sys/6(Md61SecRwLtStFwdBkwdCalib_TrgtPosArray_write) -> Md61SecRwLtStFwdBkwdCalib_TrgtPosArray/1
  Md61Md62CalibSet_Cal_sys/7(Md61SecRwLtStLgrstInwdOtwdTrgtPosCalib_TrgtPosArray_write) -> Md61SecRwLtStLgrstInwdOtwdTrgtPosCalib_TrgtPosArray/1
  Md61Md62CalibSet_Cal_sys/8(Md61SecRwLtStLgrstUpwdDnwdTrgtPosCalib_TrgtPosArray_write) -> Md61SecRwLtStLgrstUpwdDnwdTrgtPosCalib_TrgtPosArray/1
  Md61Md62CalibSet_Cal_sys/9(Md61ThdRwLtStBkReclnUpwdDnwdTrgtPosCalib_TrgtPosArray_write) -> Md61ThdRwLtStBkReclnUpwdDnwdTrgtPosCalib_TrgtPosArray/1
  Md61Md62CalibSet_Cal_sys/10(Md61ThdRwLtStCshnFldUpwdDnwdTrgtPos_Val_write) -> Md61ThdRwLtStCshnFldUpwdDnwdTrgtPos_Val/1
  Md61Md62CalibSet_Cal_sys/11(Md61ThdRwLtStCshnFldUpwdDnwdTrgtPosCalib_TrgtPosArray_write) -> Md61ThdRwLtStCshnFldUpwdDnwdTrgtPosCalib_TrgtPosArray/1
  Md61Md62CalibSet_Cal_sys/12(Md61ThdRwLtStFrwdBkwdPosTrgtPosCalib_TrgtPosArray_write) -> Md61ThdRwLtStFrwdBkwdPosTrgtPosCalib_TrgtPosArray/1
  Md61Md62CalibSet_Cal_sys/13(Md61ThdRwRtStCshnFldUpwdDnwdTrgtPos_Val_write) -> Md61ThdRwRtStCshnFldUpwdDnwdTrgtPos_Val/1
  Md61Md62CalibSet_Cal_sys/14(Md62PassStBkReclnTrgtPos_Val_write) -> Md62PassStBkReclnTrgtPos_Val/1
  Md61Md62CalibSet_Cal_sys/15(Md62PassStBkReclnTrgtPosCalib_TrgtPosArray_write) -> Md62PassStBkReclnTrgtPosCalib_TrgtPosArray/1
  Md61Md62CalibSet_Cal_sys/16(Md62PassStCshnFldTrgtPosCalib_TrgtPosArray_write) -> Md62PassStCshnFldTrgtPosCalib_TrgtPosArray/1
  Md61Md62CalibSet_Cal_sys/17(Md62PassStFwdBkwdTrgtPosCalib_TrgtPosArray_write) -> Md62PassStFwdBkwdTrgtPosCalib_TrgtPosArray/1
  Md61Md62CalibSet_Cal_sys/18(Md62SecRwLtStBkReclnTrgtPosCalib_TrgtPosArray_write) -> Md62SecRwLtStBkReclnTrgtPosCalib_TrgtPosArray/1
  Md61Md62CalibSet_Cal_sys/19(Md62SecRwLtStCushFrntTrgtPosCalib_TrgtPosArray_write) -> Md62SecRwLtStCushFrntTrgtPosCalib_TrgtPosArray/1
  Md61Md62CalibSet_Cal_sys/20(Md62SecRwLtStFwdBkwdCalib_TrgtPosArray_write) -> Md62SecRwLtStFwdBkwdCalib_TrgtPosArray/1
  Md61Md62CalibSet_Cal_sys/21(Md62SecRwLtStLgrstInwdOtwdTrgtPosCalib_TrgtPosArray_write) -> Md62SecRwLtStLgrstInwdOtwdTrgtPosCalib_TrgtPosArray/1
  Md61Md62CalibSet_Cal_sys/22(Md62SecRwLtStLgrstUpwdDnwdTrgtPosCalib_TrgtPosArray_write) -> Md62SecRwLtStLgrstUpwdDnwdTrgtPosCalib_TrgtPosArray/1
  Md61Md62CalibSet_Cal_sys/23(Md62ThdRwLtStBkReclnUpwdDnwdTrgtPosCalib_TrgtPosArray_write) -> Md62ThdRwLtStBkReclnUpwdDnwdTrgtPosCalib_TrgtPosArray/1
  Md61Md62CalibSet_Cal_sys/24(Md62ThdRwLtStCshnFldUpwdDnwdTrgtPos_Val_write) -> Md62ThdRwLtStCshnFldUpwdDnwdTrgtPos_Val/1
  Md61Md62CalibSet_Cal_sys/25(Md62ThdRwLtStCshnFldUpwdDnwdTrgtPosCalib_TrgtPosArray_write) -> Md62ThdRwLtStCshnFldUpwdDnwdTrgtPosCalib_TrgtPosArray/1
  Md61Md62CalibSet_Cal_sys/26(Md62ThdRwLtStFrwdBkwdPosTrgtPosCalib_TrgtPosArray_write) -> Md62ThdRwLtStFrwdBkwdPosTrgtPosCalib_TrgtPosArray/1
  Md61Md62CalibSet_Cal_sys/27(Md62ThdRwRtStCshnFldUpwdDnwdTrgtPos_Val_write) -> Md62ThdRwRtStCshnFldUpwdDnwdTrgtPos_Val/1
  Md61Md62CalibSet_Cal_sys/28(Md61SecRwRtStBkReclnTrgtPosCalib_TrgtPosArray_write) -> Md61SecRwRtStBkReclnTrgtPosCalib_TrgtPosArray/1
  Md61Md62CalibSet_Cal_sys/29(Md61SecRwRtStCushFrntTrgtPosCalib_TrgtPosArray_write) -> Md61SecRwRtStCushFrntTrgtPosCalib_TrgtPosArray/1
  Md61Md62CalibSet_Cal_sys/30(Md61SecRwRtStFwdBkwdCalib_TrgtPosArray_write) -> Md61SecRwRtStFwdBkwdCalib_TrgtPosArray/1
  Md61Md62CalibSet_Cal_sys/31(Md61SecRwRtStLgrstInwdOtwdTrgtPosCalib_TrgtPosArray_write) -> Md61SecRwRtStLgrstInwdOtwdTrgtPosCalib_TrgtPosArray/1
  Md61Md62CalibSet_Cal_sys/32(Md61SecRwRtStLgrstUpwdDnwdTrgtPosCalib_TrgtPosArray_write) -> Md61SecRwRtStLgrstUpwdDnwdTrgtPosCalib_TrgtPosArray/1
  Md61Md62CalibSet_Cal_sys/33(Md61ThdRwRtStBkReclnUpwdDnwdTrgtPosCalib_TrgtPosArray_write) -> Md61ThdRwRtStBkReclnUpwdDnwdTrgtPosCalib_TrgtPosArray/1
  Md61Md62CalibSet_Cal_sys/34(Md61ThdRwRtStCshnFldUpwdDnwdTrgtPosCalib_TrgtPosArray_write) -> Md61ThdRwRtStCshnFldUpwdDnwdTrgtPosCalib_TrgtPosArray/1
  Md61Md62CalibSet_Cal_sys/35(Md61ThdRwRtStFrwdBkwdPosTrgtPosCalib_TrgtPosArray_write) -> Md61ThdRwRtStFrwdBkwdPosTrgtPosCalib_TrgtPosArray/1
  Md61Md62CalibSet_Cal_sys/36(Md62SecRwRtStBkReclnTrgtPosCalib_TrgtPosArray_write) -> Md62SecRwRtStBkReclnTrgtPosCalib_TrgtPosArray/1
  Md61Md62CalibSet_Cal_sys/37(Md62SecRwRtStCushFrntTrgtPosCalib_TrgtPosArray_write) -> Md62SecRwRtStCushFrntTrgtPosCalib_TrgtPosArray/1
  Md61Md62CalibSet_Cal_sys/38(Md62SecRwRtStFwdBkwdCalib_TrgtPosArray_write) -> Md62SecRwRtStFwdBkwdCalib_TrgtPosArray/1
  Md61Md62CalibSet_Cal_sys/39(Md62SecRwRtStLgrstInwdOtwdTrgtPosCalib_TrgtPosArray_write) -> Md62SecRwRtStLgrstInwdOtwdTrgtPosCalib_TrgtPosArray/1
  Md61Md62CalibSet_Cal_sys/40(Md62SecRwRtStLgrstUpwdDnwdTrgtPosCalib_TrgtPosArray_write) -> Md62SecRwRtStLgrstUpwdDnwdTrgtPosCalib_TrgtPosArray/1
  Md61Md62CalibSet_Cal_sys/41(Md62ThdRwRtStBkReclnUpwdDnwdTrgtPosCalib_TrgtPosArray_write) -> Md62ThdRwRtStBkReclnUpwdDnwdTrgtPosCalib_TrgtPosArray/1
  Md61Md62CalibSet_Cal_sys/42(Md62ThdRwRtStCshnFldUpwdDnwdTrgtPosCalib_TrgtPosArray_write) -> Md62ThdRwRtStCshnFldUpwdDnwdTrgtPosCalib_TrgtPosArray/1
  Md61Md62CalibSet_Cal_sys/43(Md62ThdRwRtStFrwdBkwdPosTrgtPosCalib_TrgtPosArray_write) -> Md62ThdRwRtStFrwdBkwdPosTrgtPosCalib_TrgtPosArray/1
  modestate32_Val/1 -> Md61Md62CalibSet_Cal_sys/97(modestate32_Val_read)
  Md61Md62CalibSet_Cal_sys/44(Md61PassStNeedFldOpn_Val_write) -> Md61PassStNeedFldOpn_Val/1
  Md61Md62CalibSet_Cal_sys/45(Md61PassStTrgtIsFld_Val_write) -> Md61PassStTrgtIsFld_Val/1
  Md61Md62CalibSet_Cal_sys/46(Md61ThdRwLtStNeedFldOpn_Val_write) -> Md61ThdRwLtStNeedFldOpn_Val/1
  Md61Md62CalibSet_Cal_sys/47(Md61ThdRwLtStTrgtIsFld_Val_write) -> Md61ThdRwLtStTrgtIsFld_Val/1
  Md61Md62CalibSet_Cal_sys/48(Md61ThdRwRtStNeedFldOpn_Val_write) -> Md61ThdRwRtStNeedFldOpn_Val/1
  Md61Md62CalibSet_Cal_sys/49(Md61ThdRwRtStTrgtIsFld_Val_write) -> Md61ThdRwRtStTrgtIsFld_Val/1
  Md61Md62CalibSet_Cal_sys/50(Md62PassStNeedFldOpn_Val_write) -> Md62PassStNeedFldOpn_Val/1
  Md61Md62CalibSet_Cal_sys/51(Md62PassStTrgtIsFld_Val_write) -> Md62PassStTrgtIsFld_Val/1
  Md61Md62CalibSet_Cal_sys/52(Md62ThdRwLtStNeedFldOpn_Val_write) -> Md62ThdRwLtStNeedFldOpn_Val/1
  Md61Md62CalibSet_Cal_sys/53(Md62ThdRwLtStTrgtIsFld_Val_write) -> Md62ThdRwLtStTrgtIsFld_Val/1
  Md61Md62CalibSet_Cal_sys/54(Md62ThdRwRtStNeedFldOpn_Val_write) -> Md62ThdRwRtStNeedFldOpn_Val/1
  Md61Md62CalibSet_Cal_sys/55(Md62ThdRwRtStTrgtIsFld_Val_write) -> Md62ThdRwRtStTrgtIsFld_Val/1
  Md61Md62CalibSet_Cal_sys/56(EepMd61PassStBkReclnTrgtPos_S_Val_write) -> EepMd61PassStBkReclnTrgtPos_S_Val/1
  Md61Md62CalibSet_Cal_sys/57(EepMd61PassStCshnFldTrgtPos_S_Val_write) -> EepMd61PassStCshnFldTrgtPos_S_Val/1
  Md61Md62CalibSet_Cal_sys/58(EepMd61PassStFwdBkwdTrgtPos_S_Val_write) -> EepMd61PassStFwdBkwdTrgtPos_S_Val/1
  Md61Md62CalibSet_Cal_sys/59(EepMd61SecRwLtStBkReclnTrgtPos_S_Val_write) -> EepMd61SecRwLtStBkReclnTrgtPos_S_Val/1
  Md61Md62CalibSet_Cal_sys/60(EepMd61SecRwLtStCushFrntTrgtPos_S_Val_write) -> EepMd61SecRwLtStCushFrntTrgtPos_S_Val/1
  Md61Md62CalibSet_Cal_sys/61(EepMd61SecRwLtStFwdBkwdTrgtPos_S_Val_write) -> EepMd61SecRwLtStFwdBkwdTrgtPos_S_Val/1
  Md61Md62CalibSet_Cal_sys/62(EepMd61SecRwLtStLgrstInwdOtwdTrgtPos_S_Val_write) -> EepMd61SecRwLtStLgrstInwdOtwdTrgtPos_S_Val/1
  Md61Md62CalibSet_Cal_sys/63(EepMd61SecRwLtStLgrstUpwdDnwdTrgtPos_S_Val_write) -> EepMd61SecRwLtStLgrstUpwdDnwdTrgtPos_S_Val/1
  Md61Md62CalibSet_Cal_sys/64(EepMd61SecRwRtStBkReclnTrgtPos_S_Val_write) -> EepMd61SecRwRtStBkReclnTrgtPos_S_Val/1
  Md61Md62CalibSet_Cal_sys/65(EepMd61SecRwRtStCushFrntTrgtPos_S_Val_write) -> EepMd61SecRwRtStCushFrntTrgtPos_S_Val/1
  Md61Md62CalibSet_Cal_sys/66(EepMd61SecRwRtStFwdBkwdTrgtPos_S_Val_write) -> EepMd61SecRwRtStFwdBkwdTrgtPos_S_Val/1
  Md61Md62CalibSet_Cal_sys/67(EepMd61SecRwRtStLgrstInwdOtwdTrgtPos_S_Val_write) -> EepMd61SecRwRtStLgrstInwdOtwdTrgtPos_S_Val/1
  Md61Md62CalibSet_Cal_sys/68(EepMd61SecRwRtStLgrstUpwdDnwdTrgtPos_S_Val_write) -> EepMd61SecRwRtStLgrstUpwdDnwdTrgtPos_S_Val/1
  Md61Md62CalibSet_Cal_sys/69(EepMd61ThdRwLtStBkReclnTrgtPos_S_Val_write) -> EepMd61ThdRwLtStBkReclnTrgtPos_S_Val/1
  Md61Md62CalibSet_Cal_sys/70(EepMd61ThdRwLtStCshnFldTrgtPos_S_Val_write) -> EepMd61ThdRwLtStCshnFldTrgtPos_S_Val/1
  Md61Md62CalibSet_Cal_sys/71(EepMd61ThdRwLtStFwdBkwdTrgtPos_S_Val_write) -> EepMd61ThdRwLtStFwdBkwdTrgtPos_S_Val/1
  Md61Md62CalibSet_Cal_sys/72(EepMd61ThdRwRtStBkReclnTrgtPos_S_Val_write) -> EepMd61ThdRwRtStBkReclnTrgtPos_S_Val/1
  Md61Md62CalibSet_Cal_sys/73(EepMd61ThdRwRtStCshnFldTrgtPos_S_Val_write) -> EepMd61ThdRwRtStCshnFldTrgtPos_S_Val/1
  Md61Md62CalibSet_Cal_sys/74(EepMd61ThdRwRtStFwdBkwdTrgtPos_S_Val_write) -> EepMd61ThdRwRtStFwdBkwdTrgtPos_S_Val/1
  Md61Md62CalibSet_Cal_sys/75(EepMd62PassStBkReclnTrgtPos_S_Val_write) -> EepMd62PassStBkReclnTrgtPos_S_Val/1
  Md61Md62CalibSet_Cal_sys/76(EepMd62PassStCshnFldTrgtPos_S_Val_write) -> EepMd62PassStCshnFldTrgtPos_S_Val/1
  Md61Md62CalibSet_Cal_sys/77(EepMd62PassStFwdBkwdTrgtPos_S_Val_write) -> EepMd62PassStFwdBkwdTrgtPos_S_Val/1
  Md61Md62CalibSet_Cal_sys/78(EepMd62SecRwLtStBkReclnTrgtPos_S_Val_write) -> EepMd62SecRwLtStBkReclnTrgtPos_S_Val/1
  Md61Md62CalibSet_Cal_sys/79(EepMd62SecRwLtStCushFrntTrgtPos_S_Val_write) -> EepMd62SecRwLtStCushFrntTrgtPos_S_Val/1
  Md61Md62CalibSet_Cal_sys/80(EepMd62SecRwLtStFwdBkwdTrgtPos_S_Val_write) -> EepMd62SecRwLtStFwdBkwdTrgtPos_S_Val/1
  Md61Md62CalibSet_Cal_sys/81(EepMd62SecRwLtStLgrstInwdOtwdTrgtPos_S_Val_write) -> EepMd62SecRwLtStLgrstInwdOtwdTrgtPos_S_Val/1
  Md61Md62CalibSet_Cal_sys/82(EepMd62SecRwLtStLgrstUpwdDnwdTrgtPos_S_Val_write) -> EepMd62SecRwLtStLgrstUpwdDnwdTrgtPos_S_Val/1
  Md61Md62CalibSet_Cal_sys/83(EepMd62SecRwRtStBkReclnTrgtPos_S_Val_write) -> EepMd62SecRwRtStBkReclnTrgtPos_S_Val/1
  Md61Md62CalibSet_Cal_sys/84(EepMd62SecRwRtStCushFrntTrgtPos_S_Val_write) -> EepMd62SecRwRtStCushFrntTrgtPos_S_Val/1
  Md61Md62CalibSet_Cal_sys/85(EepMd62SecRwRtStFwdBkwdTrgtPos_S_Val_write) -> EepMd62SecRwRtStFwdBkwdTrgtPos_S_Val/1
  Md61Md62CalibSet_Cal_sys/86(EepMd62SecRwRtStLgrstInwdOtwdTrgtPos_S_Val_write) -> EepMd62SecRwRtStLgrstInwdOtwdTrgtPos_S_Val/1
  Md61Md62CalibSet_Cal_sys/87(EepMd62SecRwRtStLgrstUpwdDnwdTrgtPos_S_Val_write) -> EepMd62SecRwRtStLgrstUpwdDnwdTrgtPos_S_Val/1
  Md61Md62CalibSet_Cal_sys/88(EepMd62ThdRwLtStBkReclnTrgtPos_S_Val_write) -> EepMd62ThdRwLtStBkReclnTrgtPos_S_Val/1
  Md61Md62CalibSet_Cal_sys/89(EepMd62ThdRwLtStCshnFldTrgtPos_S_Val_write) -> EepMd62ThdRwLtStCshnFldTrgtPos_S_Val/1
  Md61Md62CalibSet_Cal_sys/90(EepMd62ThdRwLtStFwdBkwdTrgtPos_S_Val_write) -> EepMd62ThdRwLtStFwdBkwdTrgtPos_S_Val/1
  Md61Md62CalibSet_Cal_sys/91(EepMd62ThdRwRtStBkReclnTrgtPos_S_Val_write) -> EepMd62ThdRwRtStBkReclnTrgtPos_S_Val/1
  Md61Md62CalibSet_Cal_sys/92(EepMd62ThdRwRtStCshnFldTrgtPos_S_Val_write) -> EepMd62ThdRwRtStCshnFldTrgtPos_S_Val/1
  Md61Md62CalibSet_Cal_sys/93(EepMd62ThdRwRtStFwdBkwdTrgtPos_S_Val_write) -> EepMd62ThdRwRtStFwdBkwdTrgtPos_S_Val/1
  Md61Md62CalibSet_Cal_sys/94(Md61PassStBkReclnUpwdDnwdTrgtPosCalib_TrgtPosArray_write) -> Md61PassStBkReclnUpwdDnwdTrgtPosCalib_TrgtPosArray/1
  Md61Md62CalibSet_Cal_sys/95(Md61MemReq_Val_write) -> Md61MemReq_Val/1
  Md61Md62CalibSet_Cal_sys/96(Md62MemReq_Val_write) -> Md62MemReq_Val/1
  Md61Md62CalibSet_Cal_sys/97(Md61NotMem_Val_write) -> Md61NotMem_Val/1
  Md61Md62CalibSet_Cal_sys/98(Md62NotMem_Val_write) -> Md62NotMem_Val/1
